simulink model "Isothermansemibatch"  (R2018a)
settings: Solver=VariableStepAuto  StartTime=0.0  StopTime=500  RelTol=1e-3
settings Model: Creator=Mahe  LastModifiedBy=Mahe

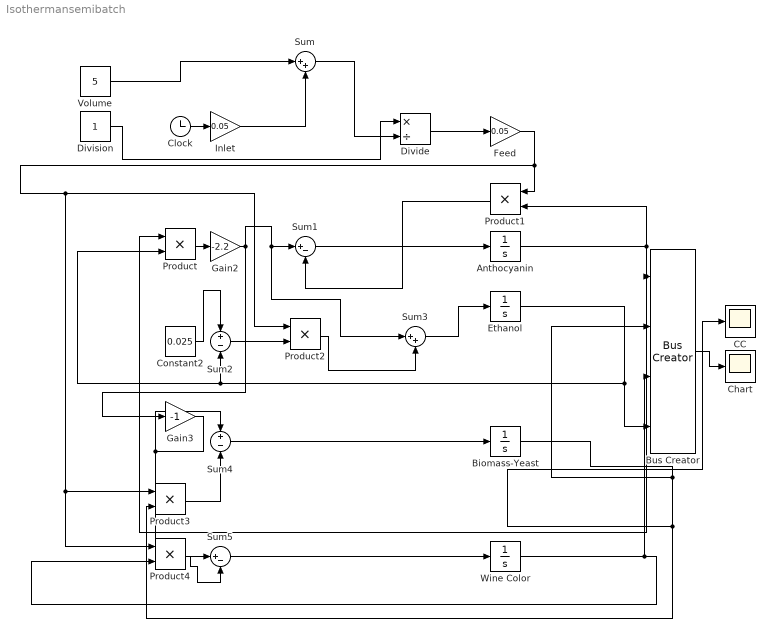
== system Isothermansemibatch ==
  Anthocyanin : Integrator  InitialCondition=0.05
  Biomass-Yeast : Integrator
  Bus Creator : BusCreator  Inputs=4
  CC : Scope
  Chart : Scope
  Clock : Clock
  Constant2 : Constant  Value=0.025
  Divide : Product  Inputs=*/
  Division : Constant
  Ethanol : Integrator
  Feed : Gain  Gain=0.05
  Gain2 : Gain  Gain=-2.2
  Gain3 : Gain  Gain=-1
  Inlet : Gain  Gain=0.05
  Product{,1..4} (5 alike) : Product
  Sum : Sum  Inputs=|++
  Sum1 : Sum  Inputs=|+-
  Sum2 : Sum  Inputs=+-
  Sum3 : Sum  Inputs=|++
  Sum4 : Sum  Inputs=+-
  Sum5 : Sum  Inputs=|+-
  Volume : Constant  Value=5
  "Wine Color " : Integrator
  wires:
  Volume/1 -> Sum/1
  Inlet/1 -> Sum/2
  Clock/1 -> Inlet/1
  Sum/1 -> Divide/2
  Division/1 -> Divide/1
  Divide/1 -> Feed/1
  Ethanol/1 -> Bus Creator/4, Sum2/2, Product/2
  Anthocyanin/1 -> Product/1, Bus Creator/1, Product1/2
  Product/1 -> Gain2/1
  Feed/1 -> Product1/1, Product4/1, Product3/1, Product2/1
  Product1/1 -> Sum1/2
  Sum1/1 -> Anthocyanin/1
  Constant2/1 -> Sum2/1
  Sum2/1 -> Product2/2
  Product2/1 -> Sum3/2
  Sum3/1 -> Ethanol/1
  Gain2/1 -> Sum3/1, Sum1/1, Gain3/1
  Gain3/1 -> Sum4/1, Sum5/1
  Biomass-Yeast/1 -> CC/1, Product3/2, Bus Creator/2
  Product3/1 -> Sum4/2
  Sum4/1 -> Biomass-Yeast/1
  "Wine Color "/1 -> Product4/2, Bus Creator/3
  Product4/1 -> Sum5/2
  Sum5/1 -> "Wine Color "/1
  Bus Creator/1 -> Chart/1
